simulink model "probleme2"  (R2024a)
settings: Solver=VariableStepAuto  StartTime=0.0  StopTime=10.0  RelTol=1e-3
settings Model: Creator=francoisdesautels  LastModifiedBy=francoisdesautels

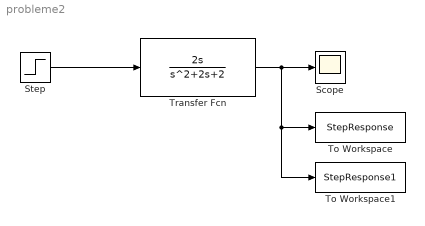
== system probleme2 ==
  Scope : Scope
  Step : Step  Time=0.01  After=10  SampleTime=0
  To Workspace : ToWorkspace  VariableName=StepResponse  SaveFormat=Timeseries  SampleTime=-1
  To Workspace1 : ToWorkspace  VariableName=StepResponse1  SaveFormat=Structure With Time  SampleTime=-1
  Transfer Fcn : TransferFcn  Numerator=[2 0]  Denominator=[1 2 2]
  wires:
  Step/1 -> Transfer Fcn/1
  Transfer Fcn/1 -> To Workspace1/1, To Workspace/1, Scope/1
